simulink model "Washing_machine_cycle of test in class on 28-10-24"  (R2024b)
settings: Solver=VariableStepAuto  StartTime=0.0  StopTime=inf  RelTol=1e-3
settings Model: Creator=hp  LastModifiedBy=madzz

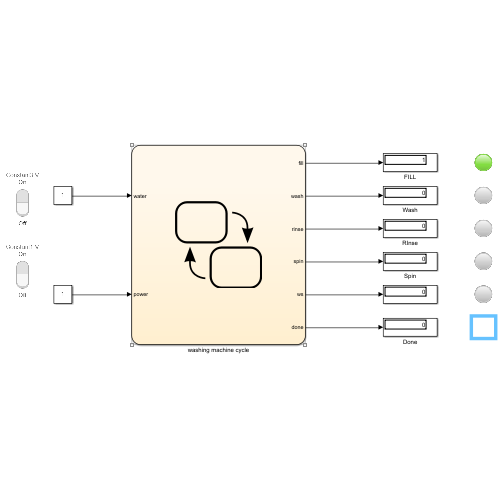
[thumbnail: Simulink's stored preview of the top-level diagram]
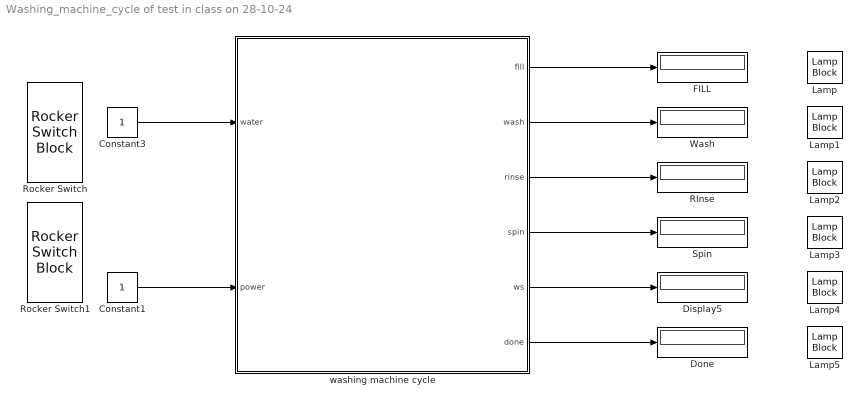
== system Washing_machine_cycle of test in class on 28-10-24 ==
  Constant1 : Constant
  Constant3 : Constant
  Display5 : Display
  Done : Display
  FILL : Display
  Lamp{,1..5} (6 alike) : LampBlock  LabelPosition=Hide
  RInse : Display
  Rocker Switch : RockerSwitchBlock
      settings: Values={{'Off', 'On'}, [0 1]}
  Rocker Switch1 : RockerSwitchBlock
      settings: Values={{'Off', 'On'}, [0 1]}
  Spin : Display
  Wash : Display
  washing machine cycle : Stateflow chart  TreatAsAtomicUnit=on
  wires:
  Constant3/1 -> washing machine cycle/1(water)
  Constant1/1 -> washing machine cycle/2(power)
  washing machine cycle/1(fill) -> FILL/1
  washing machine cycle/2(wash) -> Wash/1
  washing machine cycle/3(rinse) -> RInse/1
  washing machine cycle/4(spin) -> Spin/1
  washing machine cycle/5(ws) -> Display5/1
  washing machine cycle/6(done) -> Done/1

== stateflow chart Washing_machine_cycle of test in class on 28-10-24/washing machine cycle ==
  state done
    entry:
    spin=0,done=1;
  state rinse
    entry:
    wash=0,rinse=1;
  state spin
    entry:
    rinse=0,spin=1;
  state wash
    entry:
    fill=0,wash=1;
  state power_supply
  state water_supply
  state fill
    entry:
    fill=1;
  state water_indicator
    entry:
    ws=1;
  (default) -> power_supply
  fill -> wash : after(10,sec)
  wash -> rinse : after(10,sec)
  spin -> done : after(10,sec)
  rinse -> spin : after(10,sec)
  water_supply -> fill [order 1] : [water==1]
  power_supply -> water_supply : [power==1]
  water_supply -> water_indicator [order 2] : [water==1]
  data: water input; fill output; wash output; rinse output; spin output; ws output; done output; power input
